simulink model "rtwdemo_sfexprfold"  (Simulink 6.0)
settings: Solver=ode5  StartTime=0.0  StopTime=10.0  RelTol=1e-3
PreLoadFcn:
  | rtwdemo_exprfolding_data
values from neighbouring files (symbols this model uses):
  LOWER = Simulink.Parameter    [rtwdemo_exprfolding_data.m]
  T1Break = Simulink.Parameter    [rtwdemo_exprfolding_data.m]    (also in rtwdemo_paraminline_data.m)
  T1Data = Simulink.Parameter    [rtwdemo_exprfolding_data.m]    (also in rtwdemo_paraminline_data.m)
  T2Data = Simulink.Parameter    [rtwdemo_exprfolding_data.m]    (also in rtwdemo_paraminline_data.m)
  UPPER = Simulink.Parameter    [rtwdemo_exprfolding_data.m]
libraries: rtwdemowidgets x2
settings Model: Creator=The MathWorks Inc.  LastModifiedBy=batserve  ExtModeAutoUpdateStatusClock=off
settings DataIOCC: SaveOutput=off  SaveTime=off  SignalLoggingName=sigsOut
settings OptimizationCC: InlineParams=on  EnforceIntegerDowncast=off  StateBitsets=on  DataBitsets=on  UseTempVars=on
settings DebuggingCC: CheckExecutionContextPreStartOutputMsg=on  CheckExecutionContextRuntimeOutputMsg=on  SolverPrmCheckMsg=none
settings RTWCC: TLCOptions=-p0 -aWarnNonSaturatedBlocks=0  GenCodeOnly=on  GenerateReport=on  RTWVerbose=off  ProcessScript=grt_make_rtw_hook  LaunchReport=on
settings CodeAppCC: ForceParamTrailComments=on  PrefixModelToSubsysFcnNames=off  MangleLength=4
settings GRTTargetCC: MatFileLogging=off

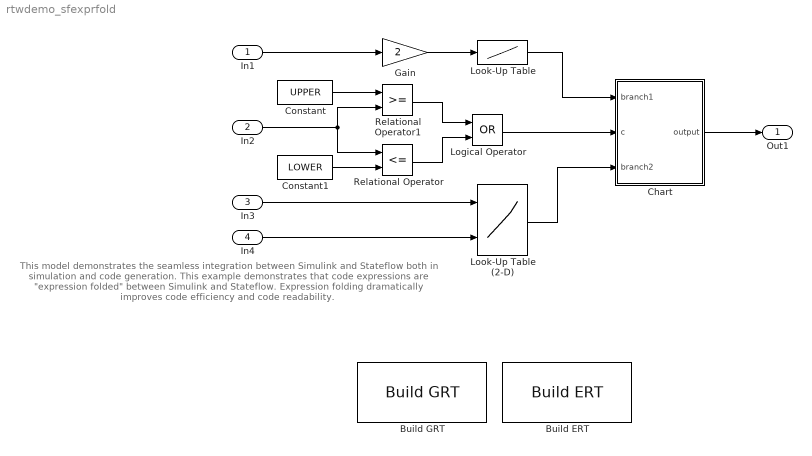
== system rtwdemo_sfexprfold ==
  note: This model demonstrates the seamless integration between Simulink and Stateflow both
      | in simulation and code generation.  This example demonstrates that code expressions
      | are "expression folded" between Simulink and Stateflow.  Expression folding dramatically
      | improves code efficiency and code readability.
  In1 : Inport  Port=1  PortDimensions=1  LatchInput=off
  In2 : Inport  Port=2  PortDimensions=1  LatchInput=off
  In3 : Inport  Port=3  PortDimensions=1  LatchInput=off
  In4 : Inport  Port=4  PortDimensions=1  LatchInput=off
  Build ERT : rtwdemowidgets/Build ERT  attrib_overrides={}
  Build GRT : rtwdemowidgets/Build GRT  attrib_overrides={}
  Chart : Stateflow chart  PropExecContextAcrossSSBoundary=on
  Constant : Constant  Value=UPPER
  Constant1 : Constant  Value=LOWER
  Gain : Gain  Gain=2  SaturateOnIntegerOverflow=on
  Logical Operator : Logic  Operator=OR
  Look-Up Table : Lookup  DialogController=Simulink.DDGSource  InputValues=T1Break  OutputValues=T1Data  SaturateOnIntegerOverflow=on
  Look-Up Table (2-D) : Lookup2D  DialogController=Simulink.DDGSource  RowIndex=T2Break  ColumnIndex=T2Break  OutputValues=T2Data  OutScaling=2^-10  InputSameDT=on
  Relational Operator : RelationalOperator  Operator=<=  InputSameDT=on
  Relational Operator1 : RelationalOperator  InputSameDT=on
  Out1 : Outport
  wires:
  Relational Operator1/1 -> Logical Operator/1
  Relational Operator/1 -> Logical Operator/2
  Logical Operator/1 -> Chart/2(c)
  Constant1/1 -> Relational Operator/2
  In1/1 -> Gain/1
  Gain/1 -> Look-Up Table/1
  Look-Up Table (2-D)/1 -> Chart/3(branch2)
  Constant/1 -> Relational Operator1/1
  In2/1 -> Relational Operator1/2, Relational Operator/1
  In3/1 -> Look-Up Table (2-D)/1
  In4/1 -> Look-Up Table (2-D)/2
  Look-Up Table/1 -> Chart/1(branch1)
  Chart/1(output) -> Out1/1

== stateflow chart Chart ==
  note: This chart is acting as an if-else condition.
      | Using a Simulink switch or if-action block
      | results in virtually identical code.
  (junction 5) -> (junction 4) : [c]{output = branch1;}
  (default) -> (junction 5)
  (junction 5) -> (junction 4) : {output = branch2;}
  data: branch1 input double size=1; c input boolean size=1; branch2 input double size=1; output output double size=1
